simulink model "fuelCycle"  (R2023b)
settings: Solver=VariableStepAuto  StartTime=0.0  StopTime=sim_time  RelTol=1e-4
values from neighbouring files (symbols this model uses):
  AF = 0.90    (= 0.9)    [FC_scenario_inputData.m]    (also in inputData.m = 70)
  eta2 = 0.95    [FC_scenario_inputData.m]    (also in inputData.m)
  f51 = 0.33    [FC_scenario_inputData.m]    (also in inputData.m)
  f53 = 0.33    [FC_scenario_inputData.m]    (also in inputData.m)
  f54 = 1 - f51 - f53 - f56    (= 0.3399)    [FC_scenario_inputData.m]    (also in inputData.m)
  f56 = 1e-4    (= 0.0001)    [FC_scenario_inputData.m]    (also in inputData.m)
  f96 = 0.1    [FC_scenario_inputData.m]    (also in inputData.m)
  f_dir = 0.7    [FC_scenario_inputData.m]    (also in inputData.m = 0.3)
  fp3 = 1e-4    (= 0.0001)    [FC_scenario_inputData.m]    (also in inputData.m; parametric_analysis_f_p_trap.m = f_p(i))
  fp4 = 1e-4    (= 0.0001)    [FC_scenario_inputData.m]    (also in inputData.m; parametric_analysis_f_p_trap.m = f_p(i))
  I_s_0 = 1.85    [fuelCycleSimulator.m]    (also in parametric_analysis_f_p_trap.m = 0.8; utilities.m = I_s_0 - abs(margin) + inventory_accuracy)
  lambda = 1.73e-9    (= 1.73e-09)    [FC_scenario_inputData.m]    (also in inputData.m)
  N_dot = 9.3e-7    (= 9.3e-07)    [FC_scenario_inputData.m]    (also in inputData.m)
  T1 = 1/((1 + epsi)/tau1 + lambda)    [FC_scenario_inputData.m]    (also in inputData.m)
  T12 = 1/((1 + epsi)/tau12 + lambda)    [FC_scenario_inputData.m]    (also in inputData.m)
  T2 = 1/((1 + epsi)/tau2 + lambda)    [FC_scenario_inputData.m]    (also in inputData.m)
  T3 = 1/((1 + 0)/tau3 + lambda)    [FC_scenario_inputData.m]    (also in inputData.m)
  T4 = 1/((1 + 0)/tau4 + lambda)    [FC_scenario_inputData.m]    (also in inputData.m)
  T5 = 1/((1 + epsi)/tau5 + lambda)    [FC_scenario_inputData.m]    (also in inputData.m)
  T6 = 1/((1 + epsi)/tau6 + lambda)    [FC_scenario_inputData.m]    (also in inputData.m)
  T7 = 1/((1 + epsi)/tau7 + lambda)    [FC_scenario_inputData.m]    (also in inputData.m)
  T8 = 1/((1 + epsi)/tau8 + lambda)    [FC_scenario_inputData.m]    (also in inputData.m)
  T9 = 1/((1 + epsi)/tau9 + lambda)    [FC_scenario_inputData.m]    (also in inputData.m)
  tau1 = 1.25*3600    (= 4500)    [FC_scenario_inputData.m]    (also in inputData.m)
  tau12 = 100    [FC_scenario_inputData.m]    (also in inputData.m)
  tau2 = 1*24*3600    (= 86400)    [FC_scenario_inputData.m]    (also in inputData.m)
  tau3 = 1000    [FC_scenario_inputData.m]    (also in inputData.m)
  tau4 = 1000    [FC_scenario_inputData.m]    (also in inputData.m)
  tau5 = 1000    [FC_scenario_inputData.m]    (also in inputData.m)
  tau6 = 3600    [FC_scenario_inputData.m]    (also in inputData.m)
  tau7 = 600    [FC_scenario_inputData.m]    (also in inputData.m)
  tau8 = 0.1*3600    (= 360)    [FC_scenario_inputData.m]    (also in inputData.m = 3600)
  tau9 = 0.9*3600    (= 3240)    [FC_scenario_inputData.m]    (also in inputData.m = 10800)
  TBE = 0.02    [FC_scenario_inputData.m]    (also in inputData.m; parametric_analysis_f_p_trap.m = TBE_array(j); parametric_analysis_trapping.m)
  TBR = 1.096    [fuelCycleSimulator.m]    (also in parametric_analysis_f_p_trap.m = 1.048; parametric_analysis_trapping.m = 1.06; utilities.m = TBR_start)
libraries: spsMeanLib x7, arc x2
settings Model: Creator=smesc  LastModifiedBy=meschini
settings SolverCC: InitialStep=1e-4  ShapePreserveControl=EnableAll
settings OptimizationCC: ReuseModelBlockBuffer=off
settings ModelReferenceCC: EnableRefExpFcnMdlSchedulingChecks=on

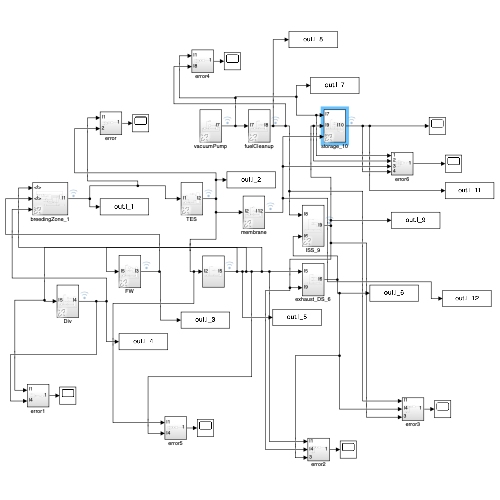
[thumbnail: Simulink's stored preview of the top-level diagram]
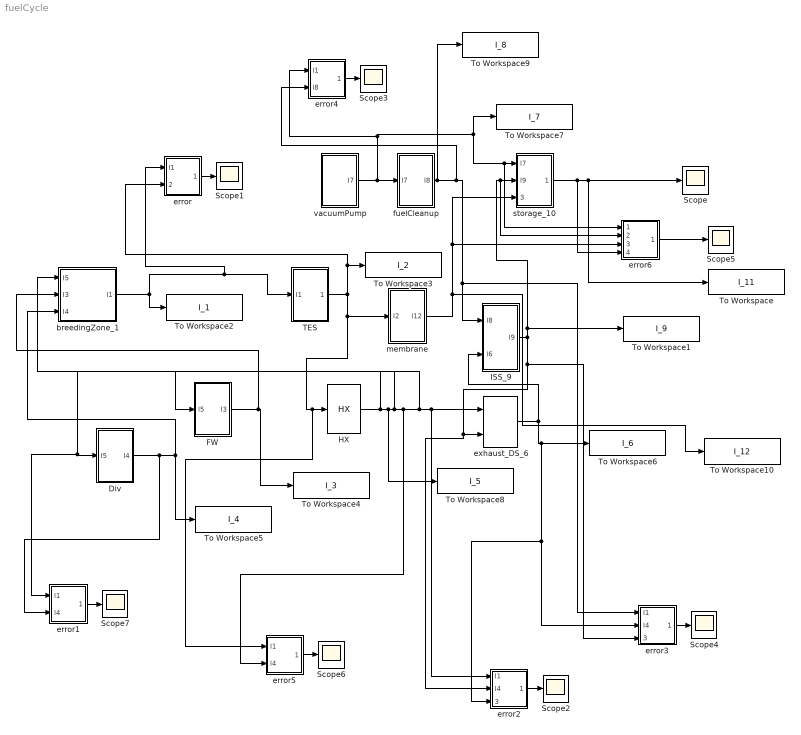
== system fuelCycle ==
  Div : Subsystem  AncestorBlock=arc/divertor_4
      settings: LibrarySourceBlock=arc/divertor_4
  FW : Subsystem  AncestorBlock=arc/FW_3
      settings: LibrarySourceBlock=arc/FW_3
  HX : arc/HX  Tag=HX  SystemSampleTime=-1  VariantActivationTime=update diagram  AllowFlexibleInterface=on  Latency=0  AutoFrameSizeCalculation=off
  ISS_9 : Subsystem  AncestorBlock=arc/ISS_9
      settings: LibrarySourceBlock=arc/ISS_9
  Scope{,1..7} (8 alike) : Scope
  TES : Subsystem  AncestorBlock=arc/TES_2
      settings: LibrarySourceBlock=arc/TES_2
  To Workspace : ToWorkspace  VariableName=I_11  SampleTime=-1
  To Workspace1 : ToWorkspace  VariableName=I_9  SampleTime=-1
  To Workspace10 : ToWorkspace  VariableName=I_12  SampleTime=-1
  To Workspace2 : ToWorkspace  VariableName=I_1  SampleTime=-1
  To Workspace3 : ToWorkspace  VariableName=I_2  SampleTime=-1
  To Workspace4 : ToWorkspace  VariableName=I_3  SampleTime=-1
  To Workspace5 : ToWorkspace  VariableName=I_4  SampleTime=-1
  To Workspace6 : ToWorkspace  VariableName=I_6  SampleTime=-1
  To Workspace7 : ToWorkspace  VariableName=I_7  SampleTime=-1
  To Workspace8 : ToWorkspace  VariableName=I_5  SampleTime=-1
  To Workspace9 : ToWorkspace  VariableName=I_8  SampleTime=-1
  breedingZone_1 : Subsystem  AncestorBlock=arc/breedingZone_1
      settings: LibrarySourceBlock=arc/breedingZone_1
  error : Subsystem
  error1 : Subsystem
  error2 : Subsystem
  error3 : Subsystem
  error4 : Subsystem
  error5 : Subsystem
  error6 : Subsystem
  exhaust_DS_6 : arc/exhaust_DS  SystemSampleTime=-1  VariantActivationTime=update diagram  AllowFlexibleInterface=on  Latency=0  AutoFrameSizeCalculation=off
      link override Gain: Gain=f56/tau5
  fuelCleanup : Subsystem  AncestorBlock=arc/fuelCleanUp
  membrane : Subsystem  AncestorBlock=arc/fuelCleanUp_8
      settings: LibrarySourceBlock=arc/fuelCleanUp_8
  storage_10 : Subsystem  AncestorBlock=arc/storage_10
      settings: LibrarySourceBlock=arc/storage_10
  vacuumPump : Subsystem  AncestorBlock=arc/pump_7
      settings: LibrarySourceBlock=arc/pump_7
  wires:
  breedingZone_1/1(I1) -> error/1(I1), TES/1(I1), To Workspace2/1
  storage_10/1(I10) -> error6/4(Input3), To Workspace/1, Scope/1
  FW/1(I3) -> breedingZone_1/2(I3), To Workspace4/1
  Div/1(I4) -> error1/2(I4), breedingZone_1/3(I4), To Workspace5/1
  membrane/1(I12) -> To Workspace10/1, storage_10/3(I12), error6/3(Input2)
  error/1(Output) -> Scope1/1
  fuelCleanup/1(I8) -> To Workspace9/1, error4/2(I8), error3/1(I1), ISS_9/1(I8)
  vacuumPump/1(I7) -> error4/1(I1), To Workspace7/1, error6/1(Input), storage_10/1(I7), fuelCleanup/1(I7)
  exhaust_DS_6/1 -> ISS_9/2(I6), error3/2(I4), error2/3(Input), To Workspace6/1
  ISS_9/1(I9) -> error3/3(Input), error2/2(I4), exhaust_DS_6/2, error6/2(Input1), storage_10/2(I9), To Workspace1/1
  HX/1 -> FW/1(I5), To Workspace8/1, error5/2(I4), error1/1(I1), Div/1(I5), error2/1(I1), exhaust_DS_6/1, breedingZone_1/1(I5)
  TES/1(Output) -> error/2(In2), To Workspace3/1, membrane/1(I2), error5/1(I1), HX/1
  error1/1(Output) -> Scope7/1
  error2/1(Output) -> Scope2/1
  error3/1(Output) -> Scope4/1
  error4/1(Output) -> Scope3/1
  error5/1(Output) -> Scope6/1
  error6/1(Output) -> Scope5/1

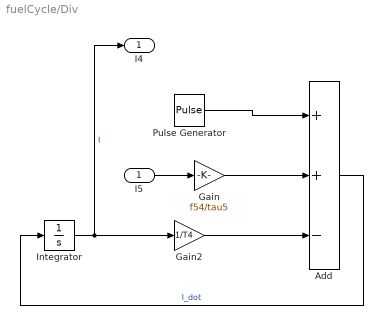
== system fuelCycle/Div ==
  I5 : Inport
  Add : Sum  Inputs=++-
  Gain : Gain  Gain=f54/tau5
  Gain2 : Gain  Gain=1/T4
  Integrator : Integrator
  Pulse Generator : DiscretePulseGenerator  PulseType=Time based  Amplitude=fp4*N_dot/TBE  Period=1800  PulseWidth=AF
  I4 : Outport
  wires:
  Pulse Generator/1 -> Add/1
  Gain/1 -> Add/2
  Integrator/1 -> Gain2/1, I4/1  "I"
  Add/1 -> Integrator/1  "I_dot"
  Gain2/1 -> Add/3
  I5/1 -> Gain/1

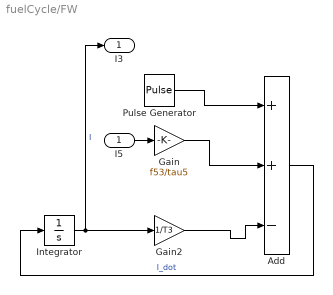
== system fuelCycle/FW ==
  I5 : Inport
  Add : Sum  Inputs=++-
  Gain : Gain  Gain=f53/tau5
  Gain2 : Gain  Gain=1/T3
  Integrator : Integrator
  Pulse Generator : DiscretePulseGenerator  PulseType=Time based  Amplitude=fp3*N_dot/TBE  Period=1800  PulseWidth=AF
  I3 : Outport
  wires:
  Gain2/1 -> Add/3
  Pulse Generator/1 -> Add/1
  Integrator/1 -> I3/1, Gain2/1  "I"
  Add/1 -> Integrator/1  "I_dot"
  Gain/1 -> Add/2
  I5/1 -> Gain/1

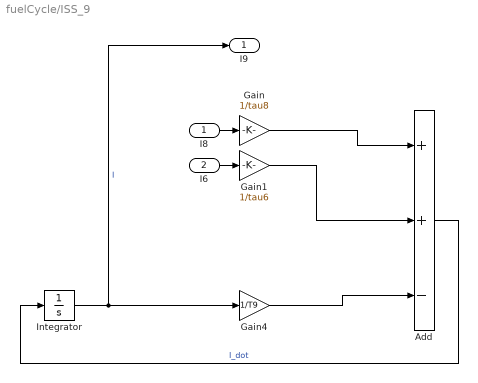
== system fuelCycle/ISS_9 ==
  I8 : Inport
  I6 : Inport  Port=2
  Add : Sum  Inputs=++-
  Gain : Gain  Gain=1/tau8
  Gain1 : Gain  Gain=1/tau6
  Gain4 : Gain  Gain=1/T9
  Integrator : Integrator
  I9 : Outport
  wires:
  I8/1 -> Gain/1
  Gain1/1 -> Add/2
  I6/1 -> Gain1/1
  Add/1 -> Integrator/1  "I_dot"
  Integrator/1 -> Gain4/1, I9/1  "I"
  Gain/1 -> Add/1
  Gain4/1 -> Add/3

== system fuelCycle/TES ==
  I1 : Inport
  Add : Sum  Inputs=+-
  Gain : Gain  Gain=1/T2
  Gain1 : Gain  Gain=1/tau1
  Integrator : Integrator
  Output : Outport
  wires:
  Gain/1 -> Add/2
  I1/1 -> Gain1/1
  Gain1/1 -> Add/1
  Integrator/1 -> Gain/1, Output/1  "I2"
  Add/1 -> Integrator/1  "I_dot"

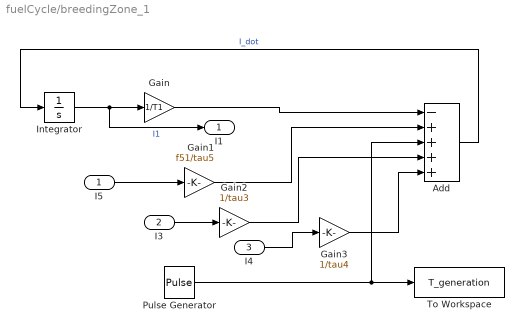
== system fuelCycle/breedingZone_1 ==
  I5 : Inport
  I3 : Inport  Port=2
  I4 : Inport  Port=3
  Add : Sum  Inputs=-++++
  Gain : Gain  Gain=1/T1
  Gain1 : Gain  Gain=f51/tau5
  Gain2 : Gain  Gain=1/tau3
  Gain3 : Gain  Gain=1/tau4
  Integrator : Integrator
  Pulse Generator : DiscretePulseGenerator  PulseType=Time based  Amplitude=N_dot * TBR  Period=1800  PulseWidth=AF
  To Workspace : ToWorkspace  VariableName=T_generation  SampleTime=-1
  I1 : Outport
  wires:
  Add/1 -> Integrator/1  "I_dot"
  Gain1/1 -> Add/2
  Integrator/1 -> Gain/1, I1/1  "I1"
  Gain/1 -> Add/1
  I5/1 -> Gain1/1
  Pulse Generator/1 -> Add/3, To Workspace/1
  I3/1 -> Gain2/1
  Gain2/1 -> Add/4
  I4/1 -> Gain3/1
  Gain3/1 -> Add/5

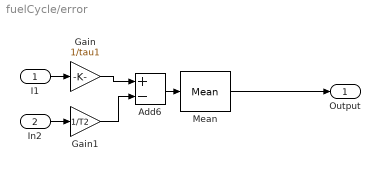
== system fuelCycle/error ==
  I1 : Inport
  In2 : Inport  Port=2
  Add6 : Sum  Inputs=+-
  Gain : Gain  Gain=1/tau1
  Gain1 : Gain  Gain=1/T2
  Mean : spsMeanLib/Mean  Freq=1/3600  Vinit=0  Ts=0
  Output : Outport
  wires:
  Gain1/1 -> Add6/2
  In2/1 -> Gain1/1
  I1/1 -> Gain/1
  Gain/1 -> Add6/1
  Add6/1 -> Mean/1
  Mean/1 -> Output/1

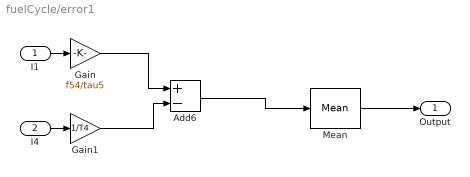
== system fuelCycle/error1 ==
  I1 : Inport
  I4 : Inport  Port=2
  Add6 : Sum  Inputs=+-
  Gain : Gain  Gain=f54/tau5
  Gain1 : Gain  Gain=1/T4
  Mean : spsMeanLib/Mean  Freq=1/3600  Vinit=0  Ts=0
  Output : Outport
  wires:
  Gain1/1 -> Add6/2
  I4/1 -> Gain1/1
  I1/1 -> Gain/1
  Gain/1 -> Add6/1
  Mean/1 -> Output/1
  Add6/1 -> Mean/1

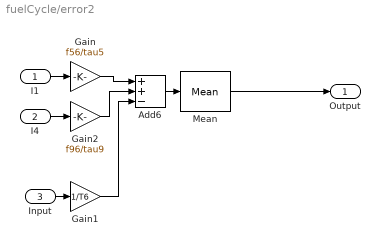
== system fuelCycle/error2 ==
  I1 : Inport
  I4 : Inport  Port=2
  Input : Inport  Port=3
  Add6 : Sum  Inputs=++-
  Gain : Gain  Gain=f56/tau5
  Gain1 : Gain  Gain=1/T6
  Gain2 : Gain  Gain=f96/tau9
  Mean : spsMeanLib/Mean  Freq=1/3600  Vinit=0  Ts=0
  Output : Outport
  wires:
  Gain1/1 -> Add6/3
  I1/1 -> Gain/1
  Gain/1 -> Add6/1
  Add6/1 -> Mean/1
  Mean/1 -> Output/1
  Input/1 -> Gain1/1
  I4/1 -> Gain2/1
  Gain2/1 -> Add6/2

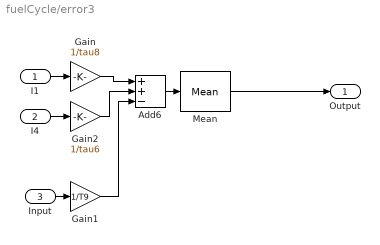
== system fuelCycle/error3 ==
  I1 : Inport
  I4 : Inport  Port=2
  Input : Inport  Port=3
  Add6 : Sum  Inputs=++-
  Gain : Gain  Gain=1/tau8
  Gain1 : Gain  Gain=1/T9
  Gain2 : Gain  Gain=1/tau6
  Mean : spsMeanLib/Mean  Freq=1/3600  Vinit=0  Ts=0
  Output : Outport
  wires:
  Gain1/1 -> Add6/3
  I1/1 -> Gain/1
  Gain/1 -> Add6/1
  Add6/1 -> Mean/1
  Mean/1 -> Output/1
  Input/1 -> Gain1/1
  I4/1 -> Gain2/1
  Gain2/1 -> Add6/2

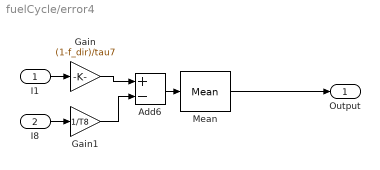
== system fuelCycle/error4 ==
  I1 : Inport
  I8 : Inport  Port=2
  Add6 : Sum  Inputs=+-
  Gain : Gain  Gain=(1-f_dir)/tau7
  Gain1 : Gain  Gain=1/T8
  Mean : spsMeanLib/Mean  Freq=1/3600  Vinit=0  Ts=0
  Output : Outport
  wires:
  Gain1/1 -> Add6/2
  I8/1 -> Gain1/1
  I1/1 -> Gain/1
  Gain/1 -> Add6/1
  Add6/1 -> Mean/1
  Mean/1 -> Output/1

== system fuelCycle/error5 ==
  I1 : Inport
  I4 : Inport  Port=2
  Add6 : Sum  Inputs=+-
  Gain : Gain  Gain=(1-eta2)/tau2
  Gain1 : Gain  Gain=1/T5
  Mean : spsMeanLib/Mean  Freq=1/3600  Vinit=0  Ts=0
  Output : Outport
  wires:
  Gain1/1 -> Add6/2
  I4/1 -> Gain1/1
  I1/1 -> Gain/1
  Gain/1 -> Add6/1
  Add6/1 -> Mean/1
  Mean/1 -> Output/1

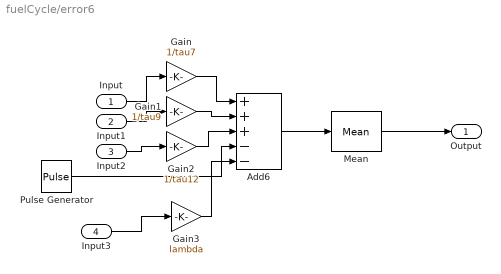
== system fuelCycle/error6 ==
  Input : Inport
  Input1 : Inport  Port=2
  Input2 : Inport  Port=3
  Input3 : Inport  Port=4
  Add6 : Sum  Inputs=+++--
  Gain : Gain  Gain=1/tau7
  Gain1 : Gain  Gain=1/tau9
  Gain2 : Gain  Gain=1/tau12
  Gain3 : Gain  Gain=lambda
  Mean : spsMeanLib/Mean  Freq=1/3600  Vinit=0  Ts=0
  Pulse Generator : DiscretePulseGenerator  PulseType=Time based  Amplitude=N_dot/TBE  Period=1800  PulseWidth=AF
  Output : Outport
  wires:
  Add6/1 -> Mean/1
  Mean/1 -> Output/1
  Gain/1 -> Add6/1
  Input/1 -> Gain/1
  Input1/1 -> Gain1/1
  Input2/1 -> Gain2/1
  Gain1/1 -> Add6/2
  Gain2/1 -> Add6/3
  Pulse Generator/1 -> Add6/4
  Input3/1 -> Gain3/1
  Gain3/1 -> Add6/5

== system fuelCycle/fuelCleanup ==
  I7 : Inport
  Add : Sum  Inputs=+-
  Gain : Gain  Gain=(1-f_dir)/tau7
  Gain1 : Gain  Gain=1/T8
  Integrator : Integrator
  I8 : Outport
  wires:
  I7/1 -> Gain/1
  Gain1/1 -> Add/2
  Add/1 -> Integrator/1  "I_dot"
  Integrator/1 -> Gain1/1, I8/1  "I"
  Gain/1 -> Add/1

== system fuelCycle/membrane ==
  I2 : Inport
  Add : Sum  Inputs=+-
  Gain : Gain  Gain=eta2/tau2
  Gain1 : Gain  Gain=1/T12
  Integrator : Integrator
  I12 : Outport
  wires:
  I2/1 -> Gain/1
  Gain1/1 -> Add/2
  Add/1 -> Integrator/1  "I_dot"
  Integrator/1 -> Gain1/1, I12/1  "I"
  Gain/1 -> Add/1

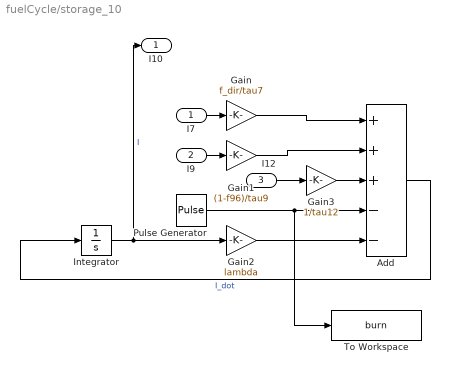
== system fuelCycle/storage_10 ==
  I7 : Inport
  I9 : Inport  Port=2
  I12 : Inport  Port=3
  Add : Sum  Inputs=+++--
  Gain : Gain  Gain=f_dir/tau7
  Gain1 : Gain  Gain=(1-f96)/tau9
  Gain2 : Gain  Gain=lambda
  Gain3 : Gain  Gain=1/tau12
  Integrator : Integrator  InitialCondition=I_s_0
  Pulse Generator : DiscretePulseGenerator  PulseType=Time based  Amplitude=N_dot/TBE  Period=1800  PulseWidth=AF
  To Workspace : ToWorkspace  VariableName=burn  SampleTime=-1
  I10 : Outport
  wires:
  Integrator/1 -> Gain2/1, I10/1  "I"
  I9/1 -> Gain1/1
  Add/1 -> Integrator/1  "I_dot"
  Gain2/1 -> Add/5
  I7/1 -> Gain/1
  Gain1/1 -> Add/2
  Gain/1 -> Add/1
  Pulse Generator/1 -> To Workspace/1, Add/4
  I12/1 -> Gain3/1
  Gain3/1 -> Add/3

== system fuelCycle/vacuumPump ==
  Add : Sum  Inputs=+-
  Gain : Gain  Gain=1/T7
  Integrator : Integrator
  Pulse Generator : DiscretePulseGenerator  PulseType=Time based  Amplitude=(1-TBE-fp3-fp4)*N_dot/TBE  Period=1800  PulseWidth=AF
  I7 : Outport
  wires:
  Gain/1 -> Add/2
  Integrator/1 -> Gain/1, I7/1  "I7"
  Pulse Generator/1 -> Add/1
  Add/1 -> Integrator/1  "I_dot"
